simulink model "validity_mc"  (R2021b)
settings: Solver=FixedStepAuto  StartTime=0.0  StopTime=10.0  RelTol=1e-3
undefined symbols (not defined in the file): sldvsubsys
libraries: sldvlib x3, simulink x1
settings Model: Creator=marco  LastModifiedBy=marco
settings ConfigComp: DVMode=PropertyProving  DVMaxProcessTime=14400  DVTestSuiteOptimization=Auto  DVDetectOutOfBounds=on  DVMaxViolationSteps=5  DVModelReferenceHarness=on

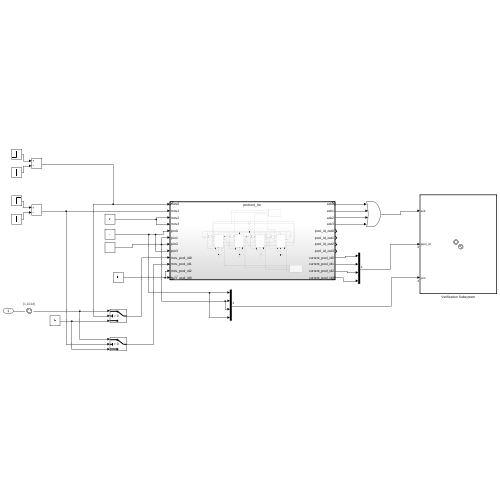
[thumbnail: Simulink's stored preview of the top-level diagram]
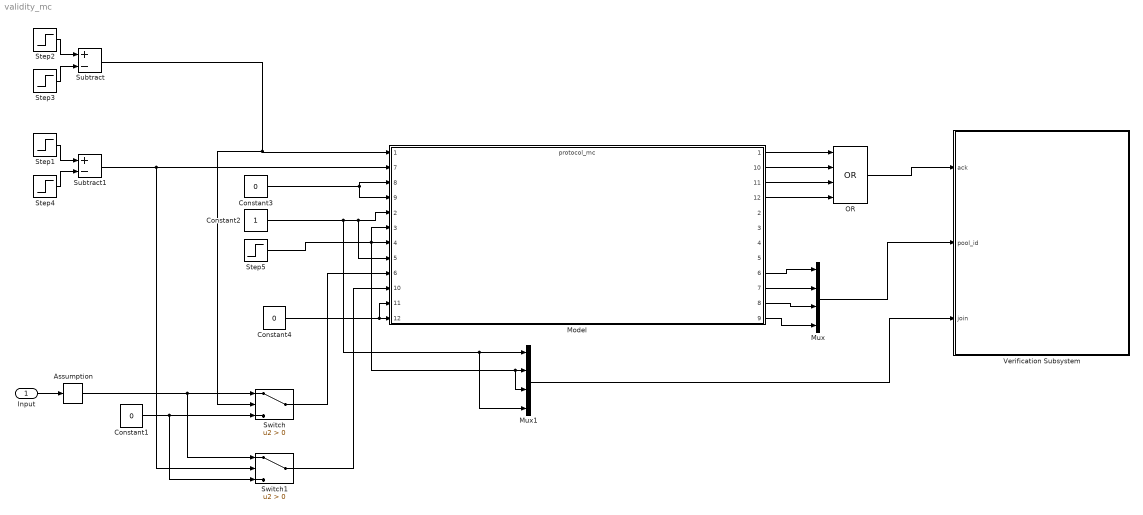
== system validity_mc ==
  Input : Inport
  Assumption : sldvlib/Objectives and Constraints/Assumption  enabled=on  customAVTBlockType=Assumption  intervals=[1,1024]  initial=off  dispValues=on  outEnabled=on
      settings: AttributesFormatString=%<intervals>  SourceProductBaseCode=SL
  Constant1 : Constant  Value=0
  Constant2 : Constant
  Constant3 : Constant  Value=0
  Constant4 : Constant  Value=0
  Model : ModelReference  ModelNameDialog=protocol_mc.slx  SimulationMode=Normal  ModelReferenceVersion=1.166
      settings: PortSchema="{\"entries\":[{\"content\":{\"sides\":[{\"content\":{\"connectorIds\":[\"In1\",\"In7\",\"In8\",\"In9\",\"In2\",\"In3\",\"In4\",\"In5\",\"In6\",\"In10\",\"In11\",\"In12\"]},\"type\":\"ConnectorPlacement.EquallySpacedRectSide\",\"uuid\":\"a8b2226d-44c9-4ce8-8c19-0bc57c3e63cc\"},{\"content\":{\"connectorIds\":[\"Out1\",\"Out10\",\"Out11\",\"Out12\",\"Out2\",\"Out3\",\"Out4\",\"Out5\",\"Out6\",\"Out7\",\"Out8\",\"Out9\"],\"side\":\"RIGHT\"},\"type\":\"ConnectorPlacement.EquallySpacedRectSide\",\"uuid\":\"6850dd4f-634c-44f8-a94c-2056f142a249\"},{\"content\":{\"connectorIds\":[],\"side\":\"TOP\"},\"type\":\"ConnectorPlacement.EquallySpacedRectSide\",\"uuid\":\"db7c17e9-d8fd-4084-957a-a148b3613c07\"}]},\"type\":\"ConnectorPlacement.EquallySpacedConnector\",\"uuid\":\"73dc548a-99fe-4585-b75f-bbc334f72eaf\"}],\"packageUris\":[\"http://schema.mathworks.com/mf0/Connector/R2020b\"],\"version\":\"1.0\"}"
  Mux : Mux
  Mux1 : Mux
  OR : Logic  Operator=OR  Inputs=4  IconShape=distinctive  AllPortsSameDT=off  OutDataTypeStr=boolean
  Step1 : Step  Time=1.6  SampleTime=.2
  Step2 : Step  Time=.2  SampleTime=.2
  Step3 : Step  Time=.4  SampleTime=.2
  Step4 : Step  Time=1.8  SampleTime=.2
  Step5 : Step  SampleTime=.2
  Subtract : Sum  Inputs=+-
  Subtract1 : Sum  Inputs=+-
  Switch : Switch  Criteria=u2 > Threshold
  Switch1 : Switch  Criteria=u2 > Threshold
  Verification Subsystem : Subsystem  Tag=VerificationSubsystem  DisableCoverage=on  LoadFcn=sldvsubsys('check')  TreatAsAtomicUnit=on  SimViewingDevice=on  mask(VerificationSubsystem){}
      mask init:
      | sldvsubsys('maskInit');
      settings: CopyFcn=sldvsubsys('copy');  OpenFcn=open_system(gcb,'force');
      settings: PreSaveFcn=|
      | set_param(gcb,'SimViewingDevice','on');
      | sldvsubsys('check');
      mask Help: helpview(fullfile(docroot,'toolbox','sldv','sldv.map'),'verificationsubsystem')
      mask Display: image(imread('sldvicon_versubsys.png','BackGroundColor',[1 1 1]),'center');
  wires:
  Step3/1 -> Subtract/2
  Step2/1 -> Subtract/1
  Subtract/1 -> Switch/2, Model/1
  Constant1/1 -> Switch1/3, Switch/3
  Switch/1 -> Model/6
  Constant2/1 -> Model/5, Model/2, Mux1/4, Mux1/1
  Step1/1 -> Subtract1/1
  Step4/1 -> Subtract1/2
  Subtract1/1 -> Model/7, Switch1/2
  Assumption/1 -> Switch1/1, Switch/1
  Constant3/1 -> Model/9, Model/8
  Switch1/1 -> Model/10
  Constant4/1 -> Model/11, Model/12
  Model/6 -> Mux/1
  Model/7 -> Mux/2
  Model/8 -> Mux/3
  Model/9 -> Mux/4
  Mux/1 -> Verification Subsystem/2(pool_id)
  Model/1 -> OR/1
  Model/10 -> OR/2
  Model/11 -> OR/3
  Model/12 -> OR/4
  OR/1 -> Verification Subsystem/1(ack)
  Mux1/1 -> Verification Subsystem/3(join)
  Step5/1 -> Model/4, Mux1/3, Mux1/2, Model/3
  Input/1 -> Assumption/1

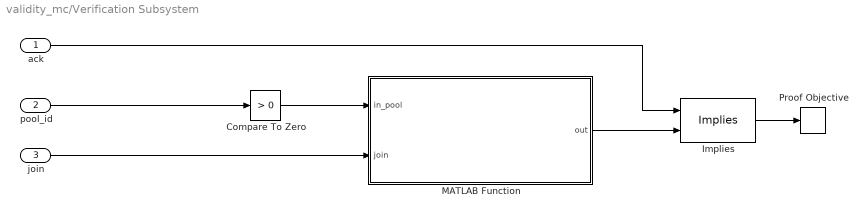
== system validity_mc/Verification Subsystem ==
  ack : Inport
  pool_id : Inport  Port=2
  join : Inport  Port=3
  Compare To Zero : simulink/Logic and Bit Operations/Compare To Zero  relop=>  OutDataTypeStr=boolean
  Implies : sldvlib/Verification Utilities/Implies
      settings: SourceProductBaseCode=SL
  MATLAB Function : MATLAB Function  TreatAsAtomicUnit=on
  Proof Objective : sldvlib/Objectives and Constraints/Proof Objective  enabled=on  customAVTBlockType=Proof Objective  intervals=true  dispValues=on  outEnabled=off  enableStopSim=off
      settings: AttributesFormatString=%<intervals>  SourceProductBaseCode=SL
  wires:
  join/1 -> MATLAB Function/2(join)
  pool_id/1 -> Compare To Zero/1
  ack/1 -> Implies/1
  Implies/1 -> Proof Objective/1
  MATLAB Function/1(out) -> Implies/2
  Compare To Zero/1 -> MATLAB Function/1(in_pool)

== matlab function validity_mc/Verification Subsystem/MATLAB Function ==
  data: in_pool input; join input; out output
function out = validity(in_pool, join)
    out = all((in_pool & join) == in_pool);
end
